simulink model "rebuilt"  (R2013b)
settings: Solver=ode45  StartTime=0.0  StopTime=100.0  RelTol=1e-6
values from neighbouring files (symbols this model uses):
  d = 1    [rebuilt_vars2.mat]
  df = 0.2    [rebuilt_vars2.mat]
  k = 2    [rebuilt_vars2.mat]
  kf = 2    [rebuilt_vars2.mat]
  m = 1    [rebuilt_vars2.mat]
settings Model: Creator=Jonas  LastModifiedBy=JNB
settings DataIOCC: SignalLoggingSaveFormat=ModelDataLogs
settings DebuggingCC: UnderspecifiedInitializationDetection=Simplified  MergeDetectMultiDrivingBlocksExec=error  MultiTaskDSMMsg=warning  MultiTaskCondExecSysMsg=none
settings RTWCC: IncludeERTFirstTime=on
settings GRTTargetCC: CodeReplacementLibrary=None  CPPClassGenCompliant=on

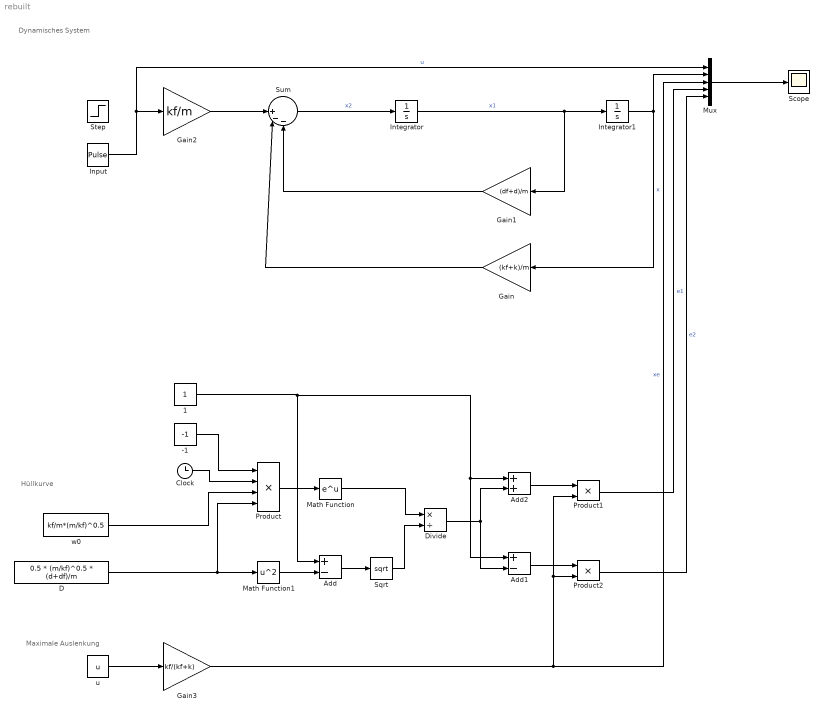
== system rebuilt ==
  note: Maximale Auslenkung
  note: Dynamisches System
  note: Hüllkurve
  -1 : Constant  Value=-1
  1 : Constant
  Add : Sum  Inputs=+-
  Add1 : Sum  Inputs=+-
  Add2 : Sum
  Clock : Clock
  D : Constant  Value=0.5 * (m/kf)^0.5 * (d+df)/m
  Divide : Product  Inputs=*/
  Gain : Gain  Gain=(kf+k)/m
  Gain1 : Gain  Gain=(df+d)/m
  Gain2 : Gain  Gain=kf/m
  Gain3 : Gain  Gain=kf/(kf+k)
  Input : DiscretePulseGenerator  PulseType=Time based  Amplitude=u  Period=40  PulseWidth=50
  Integrator : Integrator
  Integrator1 : Integrator
  Math Function : Math  SaturateOnIntegerOverflow=on
  Math Function1 : Math  Operator=square  SaturateOnIntegerOverflow=on
  Mux : Mux  Inputs=5
  Product : Product  Inputs=4
  Product1 : Product
  Product2 : Product
  Scope : Scope
      settings: ShowLegends=on
  Sqrt : Sqrt  SaturateOnIntegerOverflow=on
  Step : Step  SampleTime=0
  Sum : Sum  Inputs=||+--
  u : Constant  Value=u
  w0 : Constant  Value=kf/m*(m/kf)^0.5
  wires:
  Integrator/1 -> Gain1/1, Integrator1/1  "x1"
  Integrator1/1 -> Gain/1, Mux/2  "x"
  Gain2/1 -> Sum/1
  Sum/1 -> Integrator/1  "x2"
  Gain1/1 -> Sum/3
  Gain/1 -> Sum/2
  Mux/1 -> Scope/1
  u/1 -> Gain3/1
  Gain3/1 -> Mux/3, Product1/2, Product2/2  "xe"
  Input/1 -> Gain2/1, Mux/1  "u"
  -1/1 -> Product/1
  Clock/1 -> Product/2
  w0/1 -> Product/3
  D/1 -> Math Function1/1, Product/4
  Product/1 -> Math Function/1
  1/1 -> Add1/1, Add2/1, Add/1
  Math Function1/1 -> Add/2
  Add/1 -> Sqrt/1
  Sqrt/1 -> Divide/2
  Math Function/1 -> Divide/1
  Divide/1 -> Add2/2, Add1/2
  Add2/1 -> Product1/1
  Add1/1 -> Product2/1
  Product1/1 -> Mux/4  "e1"
  Product2/1 -> Mux/5  "e2"
